simulink model "insulatormodel"  (R2023a)
settings: Solver=VariableStepAuto  StartTime=0.0  StopTime=10.0  RelTol=1e-3
undefined symbols (not defined in the file or in its folder): gray
libraries: visionanalysis x1, dspvision x1
settings Model: Creator=Rohanlal Das  LastModifiedBy=Rohanlal Das

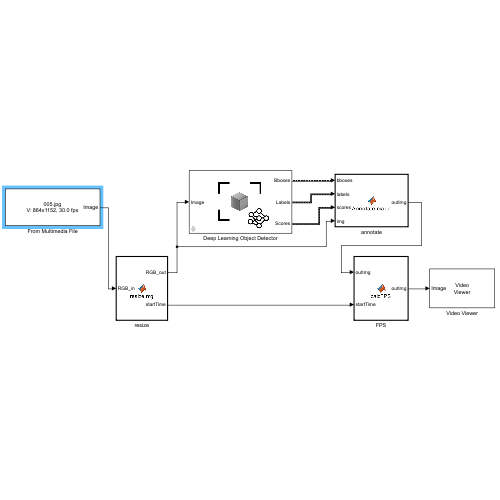
[thumbnail: Simulink's stored preview of the top-level diagram]
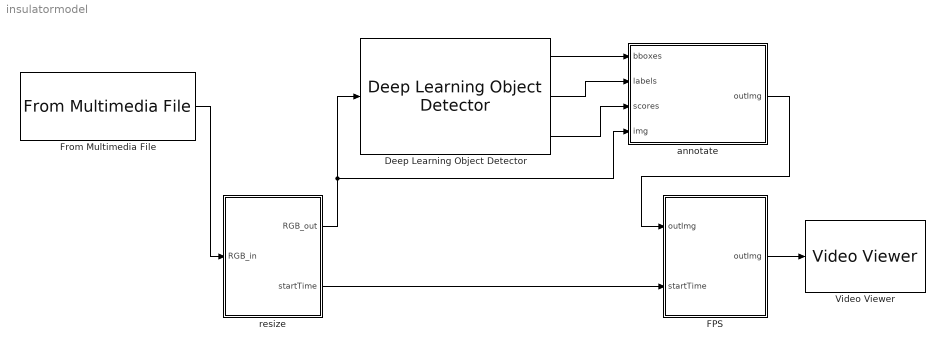
== system insulatormodel ==
  Deep Learning Object Detector : visionanalysis/Deep Learning Object Detector  Detector=Detector from MAT-file  DetectorFunction=untitled  DetectorFilePath=C:\yolo\insulatorYOLOv4.mat  MaxDetections=500  Bboxes=on  Scores=on  UseROI=off  ROI=[1 1 100 100]  Threshold=0.5  NumStrongestRegions=2000  UseMinSize=off  MinSize=[1 1]  UseMaxSize=off  MaxSize=[50 50]  ForceInterpretedSim=off
  FPS : MATLAB Function  TreatAsAtomicUnit=on
  From Multimedia File : dspvision/From Multimedia File  inputFilename=C:\yolo\insulators\images\005.jpg  readRange=[1 Inf]  loop=on  numPlays=inf  outputStreams=Video only  videoDataType=single  audioDataType=double  inheritSampleTime=on  userDefinedSampleTime=1/30  noAudioOutput=off  isIntensityVideo=off  fourcc=RGB  colorVideoFormat=One multidimensional signal  outputEOF=off  dataOrg=Column-major  audioFrameSize=1024  computeAudioFrameSize=off  outSamplingMode=Sample based
      settings: LibrarySourceBlock=audiosources/From Multimedia File
  Video Viewer : VideoViewer  colormapValue=gray(256)  FigPos=[546.6 774 857.6 545.6]
  annotate : MATLAB Function  TreatAsAtomicUnit=on
  resize : MATLAB Function  TreatAsAtomicUnit=on
  wires:
  Deep Learning Object Detector/3 -> annotate/3(scores)
  resize/2(startTime) -> FPS/2(startTime)
  From Multimedia File/1 -> resize/1(RGB_in)
  annotate/1(outImg) -> FPS/1("outImg ")
  FPS/1(outImg) -> Video Viewer/1
  resize/1(RGB_out) -> annotate/4(img), Deep Learning Object Detector/1
  Deep Learning Object Detector/2 -> annotate/2(labels)
  Deep Learning Object Detector/1 -> annotate/1(bboxes)

== matlab function insulatormodel/resize ==
  data: RGB_in input; RGB_out output; startTime output
function [RGB_out, startTime] = resizeImg(RGB_in)

    RGB_out = imresize(RGB_in,[320,320]);
    currentTime = datetime;
    startTime = [currentTime.Year currentTime.Month currentTime.Day currentTime.Hour ...
    currentTime.Minute currentTime.Second];

end

== matlab function insulatormodel/FPS ==
  data: outImg input; outImg output; startTime input
function outImg = calcFPS(outImg, startTime)
finishTime = datetime;
diffTime = seconds(finishTime-datetime(startTime));
persistent count;
if isempty(count)
count = 0;
end
persistent fps;
if isempty(fps)
fps =0;
end
fps =(count*fps +1*(1/diffTime))/(count+1);
count = count + 1;
outImg = insertText(outImg, [10 80],['FPS:' sprintf('%0.2f',fps) ], 'AnchorPoint','LeftBottom');
end

== matlab function insulatormodel/annotate ==
  data: bboxes input; labels input; scores input; img input; outImg output
function outImg = AnnotateImage(bboxes, labels,scores, img)
% Annotate detections in the image. |
if ~isempty(bboxes)
    for i = 1:numel(labels)
        labelText = sprintf('%s: %.1f%%', char(labels(i)), scores(i) * 100);
        img = insertObjectAnnotation(img, "rectangle", bboxes(i, :), labelText);
    end
end

outImg = img;

end
